simulink model "lab3"  (R2022a)
settings: Solver=VariableStepAuto  StartTime=0.0  StopTime=24 * 3600 * 10  RelTol=1e-3
values from neighbouring files (symbols this model uses):
  m = 6    [bespalov_v_m_3.m]
  n = 4    [bespalov_v_m_3.m]
settings Model: Creator=Вова  LastModifiedBy=Вова
settings SolverCC: AlgebraicLoopSolver=TrustRegion
settings DataIOCC: SaveOutput=off  SaveTime=off
settings DebuggingCC: UnconnectedInputMsg=warning  UnconnectedOutputMsg=warning  UnconnectedLineMsg=warning  SFMachineParentedDataDiag=warning  ArithmeticOperatorsInVariantConditions=warning
settings SFSimCC: SimUseLocalCustomCode=off  CustomCodeUndefinedFunction=UseInterfaceOnly
settings RTWCC: RTWUseLocalCustomCode=off  DLArmComputeVersion=19.05
settings CodeAppCC: StateflowObjectComments=on

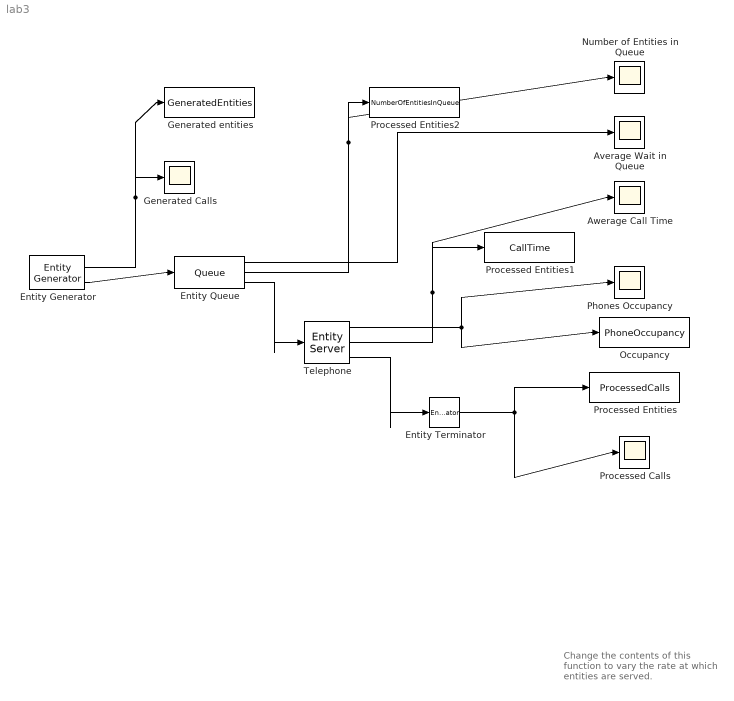
== system lab3 ==
  note: Change the contents of this function to vary the rate at which entities are served.
  Average Wait in Queue : Scope
  Awerage Call Time : Scope
  Entity Generator : EntityGenerator  OutputPortMessageModes=n,m  TimeSource=MATLAB action  IntergenerationTimeAction=|  GenerateEntityAtSimulationStart=off  NumberEntitiesDeparted=on  EntityType=Structured  EntityTypeName=Entity
      | persistent rngInit;
      | if isempty(rngInit)
      |     seed = 12345;
      |     rng(seed);
      |     rngInit = true;
      | end
      | % Pattern: Gaussian (normal) distribution
      | % m: Mean, d: Standard deviation
      | m = 270; d = 50;
      | dt = m + d * randn;
      settings: OutputPortMap=o0,o3
  Entity Queue : Queue  InputPortMessageModes=m  OutputPortMessageModes=n,n,m  Capacity=6  AverageWait=on  AverageQueueLength=on
      settings: OutputPortMap=o2,o3,o5
  Entity Terminator : EntityTerminator  InputPortMessageModes=m  NumberEntitiesArrived=on
      settings: OutputPortMap=o0
  Generated Calls : Scope
  Generated entities : ToWorkspace  VariableName=GeneratedEntities  SaveFormat=Timeseries  SampleTime=-1
  Number of Entities in Queue : Scope
  Occupancy : ToWorkspace  VariableName=PhoneOccupancy  SaveFormat=Timeseries  SampleTime=-1
  Phones Occupancy : Scope
  Processed Calls : Scope
  Processed Entities : ToWorkspace  VariableName=ProcessedCalls  SaveFormat=Timeseries  SampleTime=-1
  Processed Entities1 : ToWorkspace  VariableName=CallTime  SaveFormat=Timeseries  SampleTime=-1
  Processed Entities2 : ToWorkspace  VariableName=NumberOfEntitiesInQueue  SaveFormat=Timeseries  SampleTime=-1
  Telephone : EntityServer  InputPortMessageModes=m  OutputPortMessageModes=n,n,m  Capacity=4  ServiceTimeSource=MATLAB action  ServiceTimeAction=|  SortingAttributeName=entitySys.priority  NumberEntitiesInBlock=on  AverageWait=on
      | persistent rngInit;
      | if isempty(rngInit)
      |     seed = 567890;
      |     rng(seed);
      |     rngInit = true;
      | end
      | 
      | % Pattern: Gaussian (normal) distribution
      | % m: Mean, d: Standard deviation
      | m = 300; d = 120;
      | dt = m + d * (rand - 0.5);
      settings: OutputPortMap=o1,o4,o9
  wires:
  Telephone/3 -> Entity Terminator/1
  Entity Queue/1 -> Average Wait in Queue/1
  Entity Generator/2 -> Entity Queue/1
  Entity Queue/3 -> Telephone/1
  Telephone/2 -> Awerage Call Time/1, Processed Entities1/1
  Telephone/1 -> Occupancy/1, Phones Occupancy/1
  Entity Queue/2 -> Number of Entities in Queue/1, Processed Entities2/1
  Entity Terminator/1 -> Processed Calls/1, Processed Entities/1
  Entity Generator/1 -> Generated Calls/1, Generated entities/1
